simulink subsystem "Day3_Scenario_1"  (R2024a)
settings: Solver=VariableStepAuto  StartTime=0.0  StopTime=10.0  RelTol=1e-3
undefined symbols (not defined in the file): left_first_line_point_x, right_first_line_point_x
libraries: CarMaker4SL x6, slpidlib x1
settings Model: Creator=junhyung.cha  LastModifiedBy=User

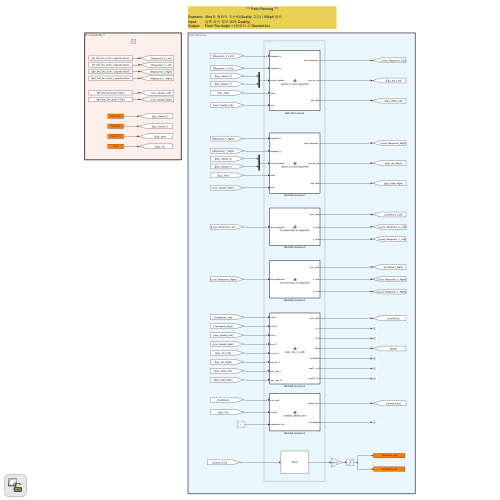
[thumbnail: Simulink's stored preview of the top-level diagram]
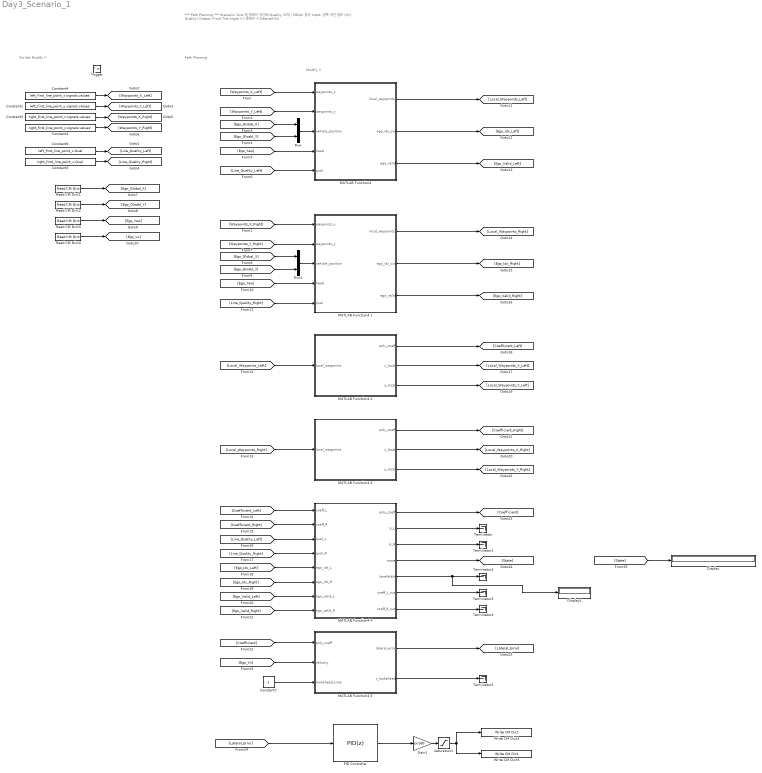
== system Day3_Scenario_1 ==
  note: Path Planning
  note: Do Not Modify !!
  note: Modify !!
  note: *** Path Planning ***
      |
      | Scenario: Sine파 형태의 곡선로(Quality 고려) / 50kph 등속
      | Input: 양쪽 차선 정보 (X/Y, Quality)
      | Output: Front Tire Angle + (종제어 시 Desired Ax)
  Trigger : TriggerPort  TriggerType=function-call  VariantControl=(inherit)
  Constant1 : Constant  Value=left_first_line_point_y.signals.values'
  Constant2 : Constant  Value=right_first_line_point_y.signals.values'
  Constant3 : Constant  Value=right_first_line_point_x.signals.values'
  Constant4 : Constant  Value=left_first_line_point_x.signals.values'
  Constant5 : Constant  Value=right_first_line_point_x.Qual
  Constant6 : Constant  Value=left_first_line_point_x.Qual
  Constant7 : Constant
  Display : Display
  Display1 : Display
  Gain1 : Gain  Gain=pi/180
  "MATLAB Function4 " : MATLAB Function  TreatAsAtomicUnit=on
  MATLAB Function4 1 : MATLAB Function  TreatAsAtomicUnit=on
  MATLAB Function4 2 : MATLAB Function  TreatAsAtomicUnit=on
  MATLAB Function4 3 : MATLAB Function  TreatAsAtomicUnit=on
  MATLAB Function4 4 : MATLAB Function  TreatAsAtomicUnit=on
  MATLAB Function4 5 : MATLAB Function  TreatAsAtomicUnit=on
  Mux : Mux  Inputs=2
  Mux1 : Mux  Inputs=2
  PID Controller : slpidlib/PID Controller  Controller=PID  Form=Parallel  TimeDomain=Discrete-time  UseExternalTs=off  SampleTime=-1  IntegratorMethod=Forward Euler  FilterMethod=Forward Euler  ControllerParametersSource=internal  P=3.0  I=0.0  UseKiTs=off  D=0.3  UseExternalDerivativeSource=off  N=20  UseFilter=on  TunerSelectOption=Transfer Function Based (PID Tuner App)  InitialConditionSource=internal  InitialConditionForIntegrator=0  InitialConditionForFilter=0  DifferentiatorICPrevScaledInput=0  ExternalReset=none  TrackingMode=off  Kt=1  LimitOutput=off  SatLimitsSource=internal  UpperSaturationLimit=inf  LowerSaturationLimit=-inf  LinearizeAsGain=on  AntiWindupMode=none  Kb=1  LimitIntegrator=off  UpperIntegratorSaturationLimit=inf  LowerIntegratorSaturationLimit=-inf  POutMin=[]  POutMax=[]  IOutMin=[]  IOutMax=[]  DOutMin=[]  DOutMax=[]  NOutMin=[]  NOutMax=[]  SumOutMin=[]  SumOutMax=[]  SaturationOutMin=[]  SaturationOutMax=[]  PParamMin=[]  PParamMax=[]  IParamMin=[]  IParamMax=[]  DParamMin=[]  DParamMax=[]  NParamMin=[]  NParamMax=[]  KbParamMin=[]  KbParamMax=[]  KtParamMin=[]  KtParamMax=[]  KbOutMin=[]  KbOutMax=[]  KtOutMin=[]  KtOutMax=[]  IntegratorOutMin=[]  IntegratorOutMax=[]  FilterOutMin=[]  FilterOutMax=[]  SumI1OutMin=[]  SumI1OutMax=[]  SumI2OutMin=[]  SumI2OutMax=[]  SumI3OutMin=[]  SumI3OutMax=[]  SumI4OutMin=[]  SumI4OutMax=[]  SumDOutMin=[]  SumDOutMax=[]  DifferentiatorOutMin=[]  DifferentiatorOutMax=[]  FilterDiffOutCoefMin=[]  FilterDiffOutCoefMax=[]  ReciprocalOutMin=[]  ReciprocalOutMax=[]  SumDenOutMin=[]  SumDenOutMax=[]  SumNumOutMin=[]  SumNumOutMax=[]  DivideOutMin=[]  DivideOutMax=[]  UdiffTsProdOutMin=[]  UdiffTsProdOutMax=[]  NTsProdOutMin=[]  NTsProdOutMax=[]  UintegralTsProdOutMin=[]  UintegralTsProdOutMax=[]  UngainTsProdOutMin=[]  UngainTsProdOutMax=[]  ClampingZeroOutDataTypeStr=Inherit: Inherit via back propagation  ClampingZeroOutMin=[]  ClampingZeroOutMax=[]  FilterDenConstantOutDataTypeStr=Inherit: Inherit via back propagation  FilterDenConstantOutMin=[]  FilterDenConstantOutMax=[]  PCopyOutDataTypeStr=Inherit: Inherit via back propagation  PCopyOutMin=[]  PCopyOutMax=[]  NCopyOutDataTypeStr=Inherit: Inherit via back propagation  NCopyOutMin=[]  NCopyOutMax=[]  IntegratorContinuousStateAttributes=''  IntegratorStateMustResolveToSignalObject=off  IntegratorRTWStateStorageClass=Auto  FilterContinuousStateAttributes=''  FilterStateMustResolveToSignalObject=off  FilterRTWStateStorageClass=Auto  ParallelPVariant=InternalParameters  IdealPVariant=Disabled  IVariant=InternalParameters  DVariant=InternalParameters  IntegratorVariant=Discrete  SatVariant=Disabled  AWVariant=Passthrough  PCopyVariant=Disabled  TRVariant=Disabled  FdbkBlocksVariant=Forward  IdealPFdbkVariant=Disabled  SatFdbkVariant=Disabled  DerivativeFilterVariant=ForwardEulerFilter  NVariant=InternalParameters  NCopyVariant=Disabled  FilterICVariant=InternalICsFilter  IntegratorICVariant=InternalICs  ExternalResetVariant=Disabled  TRSumVariant=Passthrough  SumFdbkVariant=Disabled  SumVariant=Sum_PID  TsampFilterVariant=InternalTs  TsampNgainVariant=Passthrough  TsampIntegralVariant=Disabled_SignalSpec  ExternalSaturationOutDataTypeStr=Inherit: Same as second input  DerivativeSourceVariant=ErrorSignal
  Read CM Dict1 : CarMaker4SL/Read CM Dict  xname=Car.Fr1.tx  xsync=off  xstime=Inherited
  Read CM Dict2 : CarMaker4SL/Read CM Dict  xname=Car.Fr1.ty  xsync=off  xstime=Inherited
  Read CM Dict3 : CarMaker4SL/Read CM Dict  xname=Car.Fr1.rz  xsync=off  xstime=Inherited
  Read CM Dict4 : CarMaker4SL/Read CM Dict  xname=Car.v  xsync=off  xstime=Inherited
  Saturation1 : Saturate  UpperLimit=2  LowerLimit=-2
  Terminator{,1..5} (6 alike) : Terminator
  Write CM Dict2 : CarMaker4SL/Write CM Dict  xname=Car.CFL.rz_ext  xsync=off
  Write CM Dict3 : CarMaker4SL/Write CM Dict  xname=Car.CFR.rz_ext  xsync=off
  wires:
  Constant4/1 -> [Waypoints_X_Left]
  Constant1/1 -> [Waypoints_Y_Left]
  Constant2/1 -> [Waypoints_Y_Right]
  Constant3/1 -> [Waypoints_X_Right]
  [Waypoints_X_Left] -> "MATLAB Function4 "/1(waypoints_x)
  [Waypoints_Y_Left] -> "MATLAB Function4 "/2(waypoints_y)
  Mux/1 -> "MATLAB Function4 "/3(vehicle_position)
  [Ego_Global_X] -> Mux/1
  Read CM Dict2/1 -> [Ego_Gloabl_Y]
  Read CM Dict1/1 -> [Ego_Global_X]
  [Ego_Gloabl_Y] -> Mux/2
  Read CM Dict3/1 -> [Ego_Yaw]
  [Ego_Yaw] -> "MATLAB Function4 "/4(head)
  Constant5/1 -> [Line_Quality_Right]
  Constant6/1 -> [Line_Quality_Left]
  [Line_Quality_Left] -> "MATLAB Function4 "/5(qual)
  [Line_Quality_Right] -> MATLAB Function4 1/5(qual)
  [Ego_Yaw] -> MATLAB Function4 1/4(head)
  [Ego_Gloabl_Y] -> Mux1/2
  [Ego_Global_X] -> Mux1/1
  [Waypoints_Y_Right] -> MATLAB Function4 1/2(waypoints_y)
  [Waypoints_X_Right] -> MATLAB Function4 1/1(waypoints_x)
  Mux1/1 -> MATLAB Function4 1/3(vehicle_position)
  "MATLAB Function4 "/3(ego_valid) -> [Ego_Valid_Left]
  "MATLAB Function4 "/2(ego_idx_out) -> [Ego_Idx_Left]
  "MATLAB Function4 "/1(local_waypoints_) -> [Local_Waypoints_Left]
  MATLAB Function4 1/1(local_waypoints_) -> [Local_Waypoints_Right]
  MATLAB Function4 1/2(ego_idx_out) -> [Ego_Idx_Right]
  MATLAB Function4 1/3(ego_valid) -> [Ego_Valid_Right]
  [Local_Waypoints_Left] -> MATLAB Function4 2/1(local_waypoints)
  [Local_Waypoints_Right] -> MATLAB Function4 3/1(local_waypoints)
  MATLAB Function4 2/1(poly_coeff) -> [Coefficient_Left]
  MATLAB Function4 2/2(x_local) -> [Local_Waypoints_X_Left]
  MATLAB Function4 2/3(y_local) -> [Local_Waypoints_Y_Left]
  MATLAB Function4 3/3(y_local) -> [Local_Waypoints_Y_Right]
  MATLAB Function4 3/2(x_local) -> [Local_Waypoints_X_Right]
  MATLAB Function4 3/1(poly_coeff) -> [Coefficient_Right]
  [Coefficient_Left] -> MATLAB Function4 4/1(coeff_L)
  [Coefficient_Right] -> MATLAB Function4 4/2(coeff_R)
  [Line_Quality_Left] -> MATLAB Function4 4/3(qual_L)
  [Line_Quality_Right] -> MATLAB Function4 4/4(qual_R)
  [Ego_Idx_Left] -> MATLAB Function4 4/5(ego_idx_L)
  [Ego_Idx_Right] -> MATLAB Function4 4/6(ego_idx_R)
  [Ego_Valid_Left] -> MATLAB Function4 4/7(ego_valid_L)
  [Ego_Valid_Right] -> MATLAB Function4 4/8(ego_valid_R)
  MATLAB Function4 4/1(poly_coeff) -> [Coefficient]
  MATLAB Function4 4/4(state) -> [State]
  MATLAB Function4 4/2(is_L) -> Terminator/1
  MATLAB Function4 4/3(is_R) -> Terminator1/1
  MATLAB Function4 4/6(coeff_L_out) -> Terminator3/1
  MATLAB Function4 4/5(laneWidth) -> Terminator2/1, Display1/1
  MATLAB Function4 4/7(coeff_R_out) -> Terminator4/1
  [Coefficient] -> MATLAB Function4 5/1(poly_coeff)
  Read CM Dict4/1 -> [Ego_Vx]
  [Ego_Vx] -> MATLAB Function4 5/2(velocity)
  Constant7/1 -> MATLAB Function4 5/3(lookahead_time)
  Saturation1/1 -> Write CM Dict3/1, Write CM Dict2/1
  Gain1/1 -> Saturation1/1
  MATLAB Function4 5/1(lateral_error) -> [Lateral_Error]
  MATLAB Function4 5/2(x_lookahead) -> Terminator5/1
  [Lateral_Error] -> PID Controller/1
  PID Controller/1 -> Gain1/1
  [State] -> Display/1

== matlab function Day3_Scenario_1/MATLAB Function4  ==
  settings: sampleTime=0.1
  data: waypoints_x input; waypoints_y input; local_waypoints_ output; vehicle_position input; head input; qual input; ego_idx_out output; ego_valid output
function [local_waypoints_, ego_idx_out, ego_valid] = global_to_local_waypoints(waypoints_x, waypoints_y, vehicle_position, head, qual)
    MAX_POINTS = 20; % 최대 웨이포인트 수
    local_waypoints_ = NaN(MAX_POINTS, 2); % 항상 고정 크기 반환

    % 차량 위치
    ego_x = vehicle_position(1);
    ego_y = vehicle_position(2);
    ego_yaw = head;

    % 회전 행렬 생성 (global → local)
    R = [cos(-ego_yaw), -sin(-ego_yaw);
         sin(-ego_yaw),  cos(-ego_yaw)];

    % 유효한 웨이포인트만 필터링 (qual == 1)
    valid_idx = find(qual == 1);
    if isempty(valid_idx)
        ego_idx_out = -1;
        ego_valid = false;
        return;
    end

    % 좌표 차 계산
    dx_all = waypoints_x(valid_idx) - ego_x;
    dy_all = waypoints_y(valid_idx) - ego_y;
    local_all = R * [dx_all'; dy_all'];
    local_all = local_all'; % Nx2 형식

    % 거리 계산
    dists = sqrt(dx_all.^2 + dy_all.^2);

    % 필터링 기준
    forward_idx = local_all(:,1) > 0 & dists < 15;

    filtered_local = local_all(forward_idx, :);
    filtered_dists = dists(forward_idx);
    filtered_global_idx = valid_idx(forward_idx);

    if isempty(filtered_local)
        ego_idx_out = -1;
        ego_valid = false;
        return;
    end

    % x 기준 정렬
    [~, sort_idx] = sort(filtered_local(:,1), 'ascend');
    sorted_local = filtered_local(sort_idx, :);
    sorted_dists = filtered_dists(sort_idx);
    sorted_global_idx = filtered_global_idx(sort_idx);

    % 최대 MAX_POINTS만 저장하고 나머지는 NaN
    num_points = min(size(sorted_local, 1), MAX_POINTS);
    local_waypoints_(1:num_points, :) = sorted_local(1:num_points, :);

    % 가장 가까운 웨이포인트 인덱스
    [~, min_idx] = min(sorted_dists(1:num_points));
    ego_idx_out = sorted_global_idx(min_idx);
    ego_valid = true;
end

== matlab function Day3_Scenario_1/MATLAB Function4 1 ==
  settings: sampleTime=0.1
  data: waypoints_x input; waypoints_y input; local_waypoints_ output; vehicle_position input; head input; qual input; ego_idx_out output; ego_valid output
function [local_waypoints_, ego_idx_out, ego_valid] = global_to_local_waypoints(waypoints_x, waypoints_y, vehicle_position, head, qual)
    MAX_POINTS = 20; % 최대 웨이포인트 수
    local_waypoints_ = NaN(MAX_POINTS, 2); % 항상 고정 크기 반환

    % 차량 위치
    ego_x = vehicle_position(1);
    ego_y = vehicle_position(2);
    ego_yaw = head;

    % 회전 행렬 생성 (global → local)
    R = [cos(-ego_yaw), -sin(-ego_yaw);
         sin(-ego_yaw),  cos(-ego_yaw)];

    % 유효한 웨이포인트만 필터링 (qual == 1)
    valid_idx = find(qual == 1);
    if isempty(valid_idx)
        ego_idx_out = -1;
        ego_valid = false;
        return;
    end

    % 좌표 차 계산
    dx_all = waypoints_x(valid_idx) - ego_x;
    dy_all = waypoints_y(valid_idx) - ego_y;
    local_all = R * [dx_all'; dy_all'];
    local_all = local_all'; % Nx2 형식

    % 거리 계산
    dists = sqrt(dx_all.^2 + dy_all.^2);

    % 필터링 기준
    forward_idx = local_all(:,1) > 0 & dists < 15;

    filtered_local = local_all(forward_idx, :);
    filtered_dists = dists(forward_idx);
    filtered_global_idx = valid_idx(forward_idx);

    if isempty(filtered_local)
        ego_idx_out = -1;
        ego_valid = false;
        return;
    end

    % x 기준 정렬
    [~, sort_idx] = sort(filtered_local(:,1), 'ascend');
    sorted_local = filtered_local(sort_idx, :);
    sorted_dists = filtered_dists(sort_idx);
    sorted_global_idx = filtered_global_idx(sort_idx);

    % 최대 MAX_POINTS만 저장하고 나머지는 NaN
    num_points = min(size(sorted_local, 1), MAX_POINTS);
    local_waypoints_(1:num_points, :) = sorted_local(1:num_points, :);

    % 가장 가까운 웨이포인트 인덱스
    [~, min_idx] = min(sorted_dists(1:num_points));
    ego_idx_out = sorted_global_idx(min_idx);
    ego_valid = true;
end

== matlab function Day3_Scenario_1/MATLAB Function4 2 ==
  settings: sampleTime=0.1
  data: local_waypoints input; poly_coeff output; x_local output; y_local output
function [poly_coeff, x_local, y_local] = fit_polynomial_to_waypoints(local_waypoints)
    % 최대 처리할 웨이포인트 수
    MAX_POINTS = 20;

    % 초기화
    x_local = NaN(1, MAX_POINTS);
    y_local = NaN(1, MAX_POINTS);
    poly_coeff = [0, 0, 0, 0];  % 항상 3차 다항식 형태로 초기화

    % 웨이포인트 추출
    x_points = local_waypoints(:, 1);
    y_points = local_waypoints(:, 2);

    % 유효한 포인트 (x > 0)
    valid_idx = x_points > 0;
    x_valid = x_points(valid_idx);
    y_valid = y_points(valid_idx);

    % 최대 MAX_POINTS까지만 저장
    num_valid = min(length(x_valid), MAX_POINTS);
    x_local(1:num_valid) = x_valid(1:num_valid);
    y_local(1:num_valid) = y_valid(1:num_valid);

    % 유효한 포인트가 4개 이상일 때만 3차 다항식 피팅
    if num_valid >= 4
        poly_coeff = polyfit(x_valid(1:num_valid), y_valid(1:num_valid), 3);
    end
end

== matlab function Day3_Scenario_1/MATLAB Function4 3 ==
  settings: sampleTime=0.1
  data: local_waypoints input; poly_coeff output; x_local output; y_local output
function [poly_coeff, x_local, y_local] = fit_polynomial_to_waypoints(local_waypoints)
    % 최대 처리할 웨이포인트 수
    MAX_POINTS = 20;

    % 초기화
    x_local = NaN(1, MAX_POINTS);
    y_local = NaN(1, MAX_POINTS);
    poly_coeff = [0, 0, 0, 0];  % 항상 3차 다항식 형태로 초기화

    % 웨이포인트 추출
    x_points = local_waypoints(:, 1);
    y_points = local_waypoints(:, 2);

    % 유효한 포인트 (x > 0)
    valid_idx = x_points > 0;
    x_valid = x_points(valid_idx);
    y_valid = y_points(valid_idx);

    % 최대 MAX_POINTS까지만 저장
    num_valid = min(length(x_valid), MAX_POINTS);
    x_local(1:num_valid) = x_valid(1:num_valid);
    y_local(1:num_valid) = y_valid(1:num_valid);

    % 유효한 포인트가 4개 이상일 때만 3차 다항식 피팅
    if num_valid >= 4
        poly_coeff = polyfit(x_valid(1:num_valid), y_valid(1:num_valid), 3);
    end
end

== matlab function Day3_Scenario_1/MATLAB Function4 4 ==
  settings: sampleTime=0.1
  data: coeff_L input; poly_coeff output; is_L output; is_R output; coeff_R input; qual_L input; qual_R input; ego_idx_L input; ego_idx_R input; ego_valid_L input; ego_valid_R input; state output; laneWidth output; coeff_L_out output; coeff_R_out output
function [poly_coeff, is_L, is_R, state, laneWidth, coeff_L_out, coeff_R_out] = make_line_to_path(coeff_L, coeff_R, qual_L, qual_R, ego_idx_L, ego_idx_R, ego_valid_L, ego_valid_R)
    persistent lW

    if isempty(lW)
        lW = 3.5;
        laneWidth = lW;
    end

    coeff_L_out = coeff_L;
    coeff_R_out = coeff_R;
    is_L = false;
    is_R = false;
    laneWidth = lW;

    % 양쪽 차선 모두 유효할 경우
    if ego_valid_L && ego_valid_R
        min_len = min(length(coeff_L), length(coeff_R));
        poly_coeff = (coeff_L(1:min_len) + coeff_R(1:min_len)) / 2;
        is_L = true;
        is_R = true;
        state = "Both lanes valid";

        % 실제 차선 간 폭 계산: x = 0에서의 y 좌표 차이
        % y = a*x^3 + b*x^2 + c*x + d → x=0이면 y=d
        mid_x = 5.0;
        yL = polyval(coeff_L, mid_x);
        yR = polyval(coeff_R, mid_x);
        lW = abs(yL - yR);


    % 왼쪽만 유효 → 오른쪽 가상 차선 생성
    elseif ego_valid_L
        coeff_path = coeff_L;
        coeff_path(end) = coeff_path(end) - 5;  % d항 조정
        poly_coeff = coeff_path;
        is_L = true;
        state = "Right lane missing -> Virtual right lane created";

    % 오른쪽만 유효 → 왼쪽 가상 차선 생성
    elseif ego_valid_R
        coeff_path = coeff_R;
        coeff_path(end) = coeff_path(end) + 5;  % d항 조정
        poly_coeff = coeff_path;
        is_R = true;
        state = "Left lane missing -> Virtual left lane created";

    % 둘 다 유효하지 않음
    else
        poly_coeff = [0, 0, 0, 0];
        state = "No lane detected -> Default straight path";
    end
end

== matlab function Day3_Scenario_1/MATLAB Function4 5 ==
  settings: sampleTime=0.1
  data: poly_coeff input; lateral_error output; x_lookahead output; velocity input; lookahead_time input
function [lateral_error, x_lookahead] = compute_lateral_error(poly_coeff, velocity, lookahead_time)
    % 파라미터 설정
    x_offset = 2.9;
    max_error = 2.0;
    min_error = -2.0;
    alpha = 0.15;  % 저역 필터 계수 (작을수록 더 부드러움)
    max_rate = 0.15; % 최대 변화율 제한 (m/frame)

    % persistent 저장 변수
    persistent error_buffer prev_error buffer_size

    if isempty(prev_error)
        prev_error = 0;
    end
    if isempty(buffer_size)
        buffer_size = 7;  % 최근 7개 error 누적
    end
    if isempty(error_buffer)
        error_buffer = zeros(1, buffer_size);
    end

    % lookahead 계산
    x_lookahead = velocity * lookahead_time + x_offset;
    y_desired = polyval(poly_coeff, x_lookahead);

    % 최신 error 추가
    error_buffer = [error_buffer(2:end), y_desired];

    % 중앙값 기반 보간 (튀는 값에 강함)
    median_error = median(error_buffer);

    % 저역 필터 적용
    smooth_error = alpha * median_error + (1 - alpha) * prev_error;

    % 변화율 제한 적용
    delta = smooth_error - prev_error;
    if abs(delta) > max_rate
        delta = sign(delta) * max_rate;
    end
    limited_error = prev_error + delta;

    % 제한 적용
    lateral_error = min(max(limited_error, min_error), max_error);

    % 상태 업데이트
    prev_error = lateral_error;
end
